simulink model "me_prakt3_2"  (R2025b)
settings: Solver=VariableStepAuto  StartTime=1.0  StopTime=20.0  RelTol=1e-3
settings Model: Creator=danieltchoudovski  LastModifiedBy=danieltchoudovski

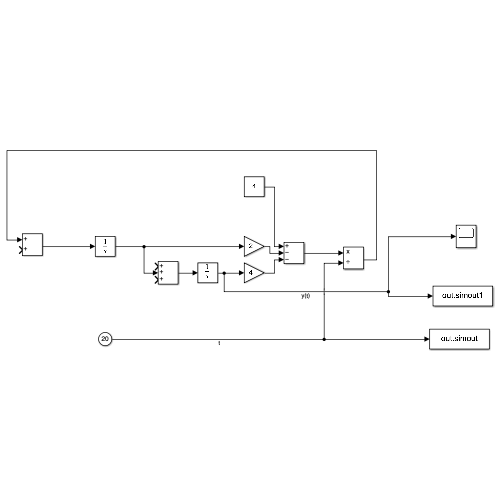
[thumbnail: Simulink's stored preview of the top-level diagram]
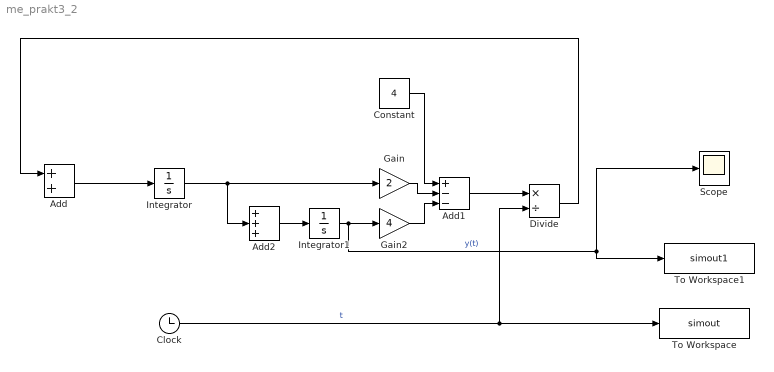
== system me_prakt3_2 ==
  Add : Sum
  Add1 : Sum  Inputs=+--
  Add2 : Sum  Inputs=+++
  Clock : Clock
  Constant : Constant  Value=4
  Divide : Product  Inputs=*/
  Gain : Gain  Gain=2
  Gain2 : Gain  Gain=4
  Integrator : Integrator  InitialCondition=1
  Integrator1 : Integrator  InitialCondition=1
  Scope : Scope
      settings: ActiveDisplayYMinimum=0.78251559957715611  ActiveDisplayYMaximum=1.375542251531537
  To Workspace : ToWorkspace  VariableName=simout  SaveFormat=Timeseries  SampleTime=-1
  To Workspace1 : ToWorkspace  VariableName=simout1  SaveFormat=Timeseries  SampleTime=-1
  wires:
  Constant/1 -> Add1/1
  Integrator/1 -> Add2/2, Gain/1
  Add/1 -> Integrator/1
  Divide/1 -> Add/1
  Clock/1 -> Divide/2, To Workspace/1  "t"
  Integrator1/1 -> To Workspace1/1, Scope/1, Gain2/1  "y(t)"
  Gain2/1 -> Add1/3
  Gain/1 -> Add1/2
  Add1/1 -> Divide/1
  Add2/1 -> Integrator1/1
